simulink model "linearizedUnicycleRobot"  (R2024b)
settings: Solver=FixedStepAuto  StartTime=0.0  StopTime=10  FixedStep=0.001  RelTol=1e-3
values from neighbouring files (symbols this model uses):
  A = [ k1*v*cos(theta) 0 -v*sin(theta) ... (first row only)    [SimRun.m]
  B = [  0    0 ... (first row only)    [SimRun.m]
  C = [1 0 0 ... (first row only)    [SimRun.m]
  D = [0 0 ... (first row only)    [SimRun.m]
  IC = [-1 1 pi/4]    [SimRun.m]
settings Model: Creator=elija  LastModifiedBy=elija

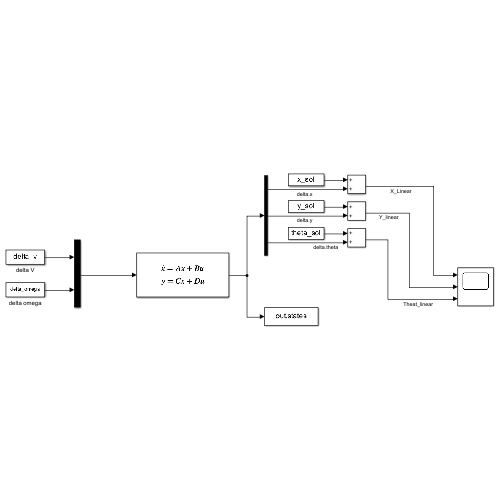
[thumbnail: Simulink's stored preview of the top-level diagram]
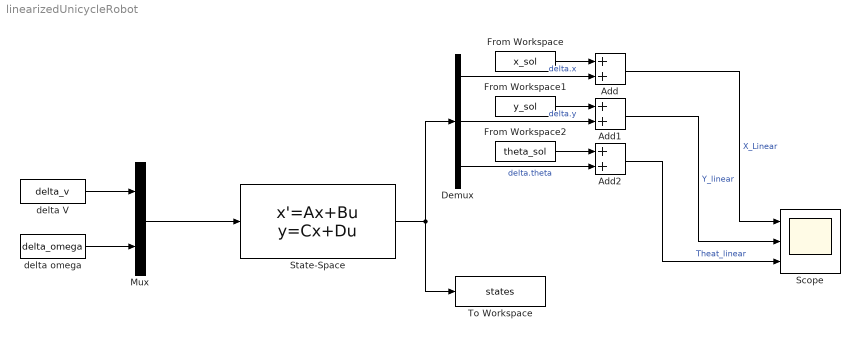
== system linearizedUnicycleRobot ==
  Add : Sum
  Add1 : Sum
  Add2 : Sum
  Demux : Demux  Outputs=3
  From Workspace : FromWorkspace  VariableName=x_sol
  From Workspace1 : FromWorkspace  VariableName=y_sol
  From Workspace2 : FromWorkspace  VariableName=theta_sol
  Mux : Mux  Inputs=2
  Scope : Scope  NumInputPorts=3
  State-Space : StateSpace  A=A  B=B  C=C  D=D  InitialCondition=IC
  To Workspace : ToWorkspace  VariableName=states  SaveFormat=Timeseries  SampleTime=-1
  delta V : FromWorkspace  VariableName=delta_v
  delta omega : FromWorkspace  VariableName=delta_omega
  wires:
  delta omega/1 -> Mux/2
  delta V/1 -> Mux/1
  Mux/1 -> State-Space/1
  State-Space/1 -> To Workspace/1, Demux/1
  Demux/1 -> Add/2  "delta.x"
  Demux/2 -> Add1/2  "delta.y"
  Demux/3 -> Add2/2  "delta.theta"
  From Workspace/1 -> Add/1
  Add/1 -> Scope/1  "X_Linear"
  From Workspace1/1 -> Add1/1
  From Workspace2/1 -> Add2/1
  Add1/1 -> Scope/2  "Y_linear"
  Add2/1 -> Scope/3  "Theat_linear"
